simulink model "SumaCoseno_6CV3"  (R2023a)
settings: Solver=FixedStepAuto  StartTime=-2*pi  StopTime=2*pi  FixedStep=pi/1500  RelTol=1e-3
libraries: dspfdesign x1, dspxfrm3 x1
settings Model: Creator=bborj  LastModifiedBy=Jorge
settings SolverCC: AlgebraicLoopSolver=TrustRegion
settings DebuggingCC: UnconnectedInputMsg=warning  UnconnectedOutputMsg=warning  UnconnectedLineMsg=warning
settings ModelReferenceCC: EnableRefExpFcnMdlSchedulingChecks=on
settings RTWCC: DLArmComputeVersion=19.05

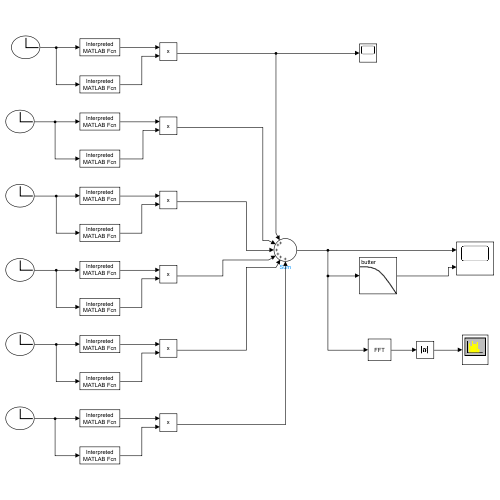
[thumbnail: Simulink's stored preview of the top-level diagram]
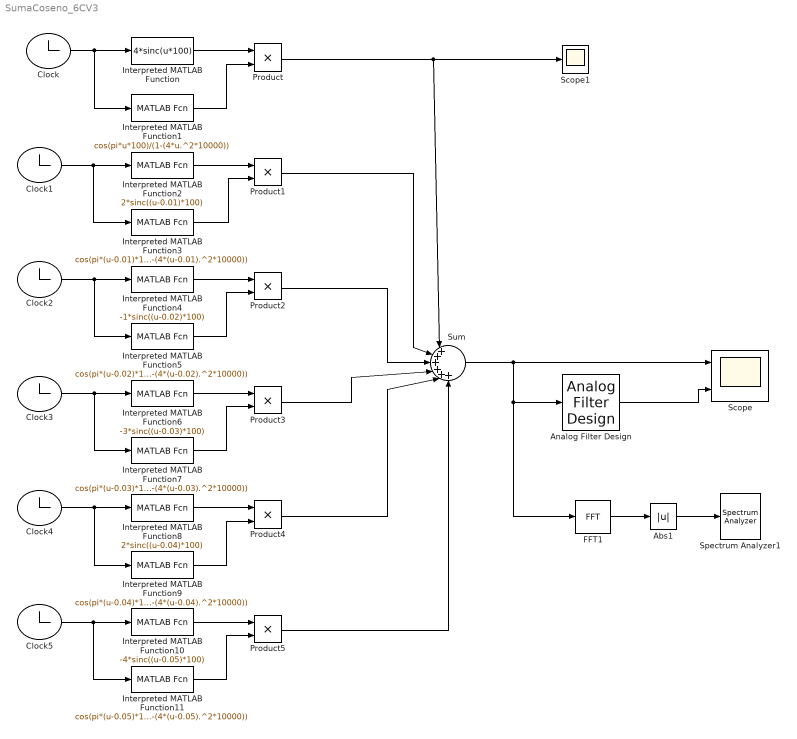
== system SumaCoseno_6CV3 ==
  Abs1 : Abs  SaturateOnIntegerOverflow=off
  Analog Filter Design : dspfdesign/Analog Filter Design  method=Butterworth  filttype=Lowpass  N=1  Wlo=2*pi*100  Whi=80  Rp=2  Rs=40
  Clock{,1..5} (6 alike) : Clock
  FFT1 : dspxfrm3/FFT  FFTImplementation=Auto  CompMethod=Table lookup  TableOpt=NEW  TableOptActive=Speed  BitRevOrder=off  Normalize=off  InheritFFTLength=on  FFTLength=64  WrapInput=on  roundingMode=Floor  overflowMode=off  firstCoeffDataTypeStr=Inherit: Same word length as input  firstCoeffLastDataTypeStr=Inherit: Same word length as input  outputMin=[]  outputMax=[]
  Interpreted MATLAB Function : MATLABFcn  MATLABFcn=4*sinc(u*100)
  Interpreted MATLAB Function1 : MATLABFcn  MATLABFcn=cos(pi*u*100)/(1-(4*u.^2*10000))
  Interpreted MATLAB Function10 : MATLABFcn  MATLABFcn=-4*sinc((u-0.05)*100)
  Interpreted MATLAB Function11 : MATLABFcn  MATLABFcn=cos(pi*(u-0.05)*100)/(1-(4*(u-0.05).^2*10000))
  Interpreted MATLAB Function2 : MATLABFcn  MATLABFcn=2*sinc((u-0.01)*100)
  Interpreted MATLAB Function3 : MATLABFcn  MATLABFcn=cos(pi*(u-0.01)*100)/(1-(4*(u-0.01).^2*10000))
  Interpreted MATLAB Function4 : MATLABFcn  MATLABFcn=-1*sinc((u-0.02)*100)
  Interpreted MATLAB Function5 : MATLABFcn  MATLABFcn=cos(pi*(u-0.02)*100)/(1-(4*(u-0.02).^2*10000))
  Interpreted MATLAB Function6 : MATLABFcn  MATLABFcn=-3*sinc((u-0.03)*100)
  Interpreted MATLAB Function7 : MATLABFcn  MATLABFcn=cos(pi*(u-0.03)*100)/(1-(4*(u-0.03).^2*10000))
  Interpreted MATLAB Function8 : MATLABFcn  MATLABFcn=2*sinc((u-0.04)*100)
  Interpreted MATLAB Function9 : MATLABFcn  MATLABFcn=cos(pi*(u-0.04)*100)/(1-(4*(u-0.04).^2*10000))
  Product{,1..5} (6 alike) : Product
  Scope : Scope  NumInputPorts=2
  Scope1 : Scope
  Spectrum Analyzer1 : SpectrumAnalyzer  WindowPosition=[2882.000000,542.000000,958.000000,508.000000,]  Visible=on  ScopeFrameLocation=window  SampleRate=477.464829275686  AxesScaling=Manual  Span=477.464829275686  StartFrequency=-238.732414637843  StopFrequency=238.732414637843  AveragingMethod=Exponential  YLimits=[-150.1392740907762402,-32.951899435865726673]  DefaultConfigurationName=spbscopes.SpectrumAnalyzerBlockCfg  IsFrequencyInputMode=0  FrequencyVectorPort=0  FrequencyVectorFromPort=0  FrequencyInputRBWPort=0  FrequencyInputRBWFromPort=0
  Sum : Sum  Inputs=|++++++
  wires:
  Clock1/1 -> Interpreted MATLAB Function3/1, Interpreted MATLAB Function2/1
  Clock/1 -> Interpreted MATLAB Function1/1, Interpreted MATLAB Function/1
  Interpreted MATLAB Function1/1 -> Product/2
  Interpreted MATLAB Function/1 -> Product/1
  Interpreted MATLAB Function2/1 -> Product1/1
  Product/1 -> Scope1/1, Sum/1
  Interpreted MATLAB Function3/1 -> Product1/2
  Clock3/1 -> Interpreted MATLAB Function7/1, Interpreted MATLAB Function6/1
  Clock2/1 -> Interpreted MATLAB Function5/1, Interpreted MATLAB Function4/1
  Interpreted MATLAB Function5/1 -> Product2/2
  Interpreted MATLAB Function4/1 -> Product2/1
  Interpreted MATLAB Function6/1 -> Product3/1
  Interpreted MATLAB Function7/1 -> Product3/2
  Clock5/1 -> Interpreted MATLAB Function10/1, Interpreted MATLAB Function11/1
  Clock4/1 -> Interpreted MATLAB Function9/1, Interpreted MATLAB Function8/1
  Interpreted MATLAB Function9/1 -> Product4/2
  Interpreted MATLAB Function8/1 -> Product4/1
  Interpreted MATLAB Function10/1 -> Product5/1
  Product4/1 -> Sum/5
  Product5/1 -> Sum/6
  Interpreted MATLAB Function11/1 -> Product5/2
  Product2/1 -> Sum/3
  Product3/1 -> Sum/4
  Product1/1 -> Sum/2
  Sum/1 -> FFT1/1, Analog Filter Design/1, Scope/1
  Analog Filter Design/1 -> Scope/2
  FFT1/1 -> Abs1/1
  Abs1/1 -> Spectrum Analyzer1/1
